simulink model "BMS_Arch_Harness_SIL"  (R2022b)
settings: configuration reference "BMS_Sw_CodeGenConfig" (kept outside this file)
undefined symbols (not defined in the file): BMS_State_Enum
settings Model: DataDictionary=BMS_Arch_DD.sldd  Creator=MAAM  LastModifiedBy=MAAM
settings ConfigSetRef: SourceName=BMS_Sw_CodeGenConfig

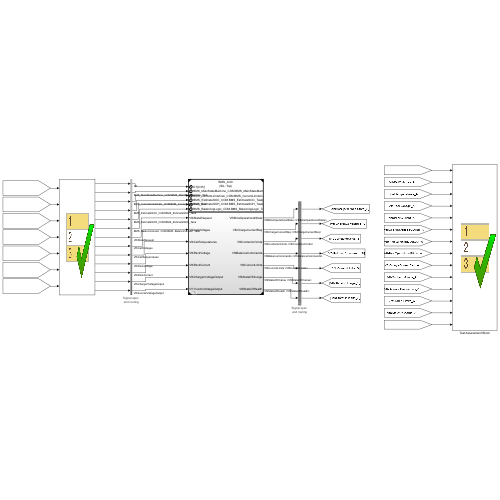
[thumbnail: Simulink's stored preview of the top-level diagram]
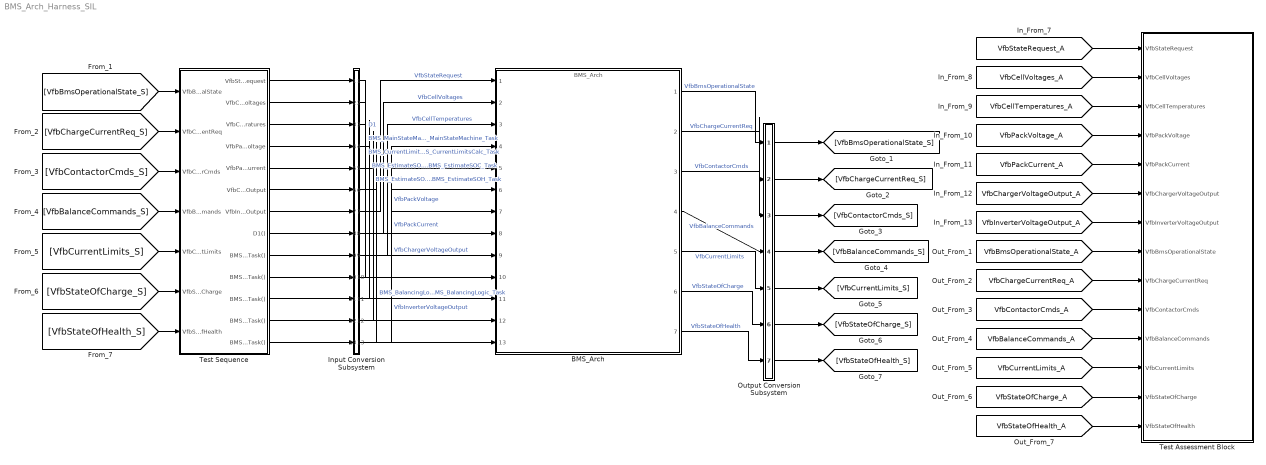
== system BMS_Arch_Harness_SIL ==
  BMS_Arch : ModelReference  ModelNameDialog=BMS_Arch  SimulationMode=Software-in-the-loop (SIL)  ScheduleRates=on  PortDiscreteRates={'',0.05;'BMS_MainStateMachine_COM.BMS_MainStateMachine_Task',0.05;'BMS_CurrentLimitsCalc_COM.BMS_CurrentLimitsCalc_Task',0.1;'BMS_EstimateSOC_COM.BMS_EstimateSOC_Task',0.2;'BMS_EstimateSOH_COM.BMS_EstimateSOH_Task',0.2;'BMS_BalancingLogic_COM.BMS_BalancingLogic_Task',0.25}  CachedPortDiscreteRates={'',0.05;'BMS_MainStateMachine_COM.BMS_MainStateMachine_Task',0.05;'BMS_CurrentLimitsCalc_COM.BMS_CurrentLimitsCalc_Task',0.1;'BMS_EstimateSOC_COM.BMS_EstimateSOC_Task',0.2;'BMS_EstimateSOH_COM.BMS_EstimateSOH_Task',0.2;'BMS_BalancingLogic_COM.BMS_BalancingLogic_Task',0.25}  AutoFillPortDiscreteRates=off  ModelEventPortInfo=P:D1[0.05][0][0],P:BMS_MainStateMachine_COM.BMS_MainStateMachine_Task[0.05][1][0],P:BMS_CurrentLimitsCalc_COM.BMS_CurrentLimitsCalc_Task[0.1][1][0],P:BMS_EstimateSOC_COM.BMS_EstimateSOC_Task[0.2][1][0],P:BMS_EstimateSOH_COM.BMS_EstimateSOH_Task[0.2][1][0],P:BMS_BalancingLogic_COM.BMS_BalancingLogic_Task[0.25][1][0]  CodeInterface=Top model  ModelReferenceVersion=1.62
  Input Conversion Subsystem : Subsystem  Tag=__SLT_ICS__  Description=|
      | Signal spec.
      | and routing
      settings: AttributesFormatString=%<Description>
  Output Conversion Subsystem : Subsystem  Tag=__SLT_OCS__  Description=|
      | Signal spec.
      | and routing
      mask init:
      | ICDictionary = get_param(bdroot, 'DataDictionary');
      | if isempty(ICDictionary)
      |    ICScope = Simulink.data.BaseWorkspace;
      | else
      |    ICScope = Simulink.data.DataDictionary(ICDictionary);
      | end
      | 
      | IC3 = Simulink.Bus.createMATLABStruct('BMS_strContactorCmds', [], [1 1], ICScope);
      settings: AttributesFormatString=%<Description>
  Test Assessment Block : Test Sequence  Tag=__SLT_ASMT__  TreatAsAtomicUnit=on
  Test Sequence : Test Sequence  TreatAsAtomicUnit=on
  wires:
  [VfbStateRequest_A] -> Test Assessment Block/1(VfbStateRequest)
  [VfbCellVoltages_A] -> Test Assessment Block/2(VfbCellVoltages)
  [VfbCellTemperatures_A] -> Test Assessment Block/3(VfbCellTemperatures)
  [VfbPackVoltage_A] -> Test Assessment Block/4(VfbPackVoltage)
  [VfbPackCurrent_A] -> Test Assessment Block/5(VfbPackCurrent)
  [VfbChargerVoltageOutput_A] -> Test Assessment Block/6(VfbChargerVoltageOutput)
  [VfbInverterVoltageOutput_A] -> Test Assessment Block/7(VfbInverterVoltageOutput)
  [VfbBmsOperationalState_A] -> Test Assessment Block/8(VfbBmsOperationalState)
  [VfbChargeCurrentReq_A] -> Test Assessment Block/9(VfbChargeCurrentReq)
  [VfbContactorCmds_A] -> Test Assessment Block/10(VfbContactorCmds)
  [VfbBalanceCommands_A] -> Test Assessment Block/11(VfbBalanceCommands)
  [VfbCurrentLimits_A] -> Test Assessment Block/12(VfbCurrentLimits)
  [VfbStateOfCharge_A] -> Test Assessment Block/13(VfbStateOfCharge)
  [VfbStateOfHealth_A] -> Test Assessment Block/14(VfbStateOfHealth)
  Test Sequence/1(VfbStateRequest) -> Input Conversion Subsystem/1(Inport_1)
  Test Sequence/2(VfbCellVoltages) -> Input Conversion Subsystem/2(Inport_2)
  Test Sequence/3(VfbCellTemperatures) -> Input Conversion Subsystem/3(Inport_3)
  Test Sequence/4(VfbPackVoltage) -> Input Conversion Subsystem/4(Inport_4)
  Test Sequence/5(VfbPackCurrent) -> Input Conversion Subsystem/5(Inport_5)
  Test Sequence/6(VfbChargerVoltageOutput) -> Input Conversion Subsystem/6(Inport_6)
  Test Sequence/7(VfbInverterVoltageOutput) -> Input Conversion Subsystem/7(Inport_7)
  Test Sequence/8(D1()) -> Input Conversion Subsystem/8(Inport_8)
  Test Sequence/9(BMS_MainStateMachine_COMBMS_MainStateMachine_Task()) -> Input Conversion Subsystem/9(Inport_9)
  Test Sequence/10(BMS_CurrentLimitsCalc_COMBMS_CurrentLimitsCalc_Task()) -> Input Conversion Subsystem/10(Inport_10)
  Test Sequence/11(BMS_EstimateSOC_COMBMS_EstimateSOC_Task()) -> Input Conversion Subsystem/11(Inport_11)
  Test Sequence/12(BMS_EstimateSOH_COMBMS_EstimateSOH_Task()) -> Input Conversion Subsystem/12(Inport_12)
  Test Sequence/13(BMS_BalancingLogic_COMBMS_BalancingLogic_Task()) -> Input Conversion Subsystem/13(Inport_13)
  [VfbBmsOperationalState_S] -> Test Sequence/1(VfbBmsOperationalState)
  [VfbChargeCurrentReq_S] -> Test Sequence/2(VfbChargeCurrentReq)
  [VfbContactorCmds_S] -> Test Sequence/3(VfbContactorCmds)
  [VfbBalanceCommands_S] -> Test Sequence/4(VfbBalanceCommands)
  [VfbCurrentLimits_S] -> Test Sequence/5(VfbCurrentLimits)
  [VfbStateOfCharge_S] -> Test Sequence/6(VfbStateOfCharge)
  [VfbStateOfHealth_S] -> Test Sequence/7(VfbStateOfHealth)
  Output Conversion Subsystem/1(Outport_1) -> [VfbBmsOperationalState_S]
  Output Conversion Subsystem/2(Outport_2) -> [VfbChargeCurrentReq_S]
  Output Conversion Subsystem/3(Outport_3) -> [VfbContactorCmds_S]
  Output Conversion Subsystem/4(Outport_4) -> [VfbBalanceCommands_S]
  Output Conversion Subsystem/5(Outport_5) -> [VfbCurrentLimits_S]
  Output Conversion Subsystem/6(Outport_6) -> [VfbStateOfCharge_S]
  Output Conversion Subsystem/7(Outport_7) -> [VfbStateOfHealth_S]
  BMS_Arch/1 -> Output Conversion Subsystem/1(Inport_1)  "VfbBmsOperationalState"
  BMS_Arch/2 -> Output Conversion Subsystem/2(Inport_2)  "VfbChargeCurrentReq"
  BMS_Arch/3 -> Output Conversion Subsystem/3(Inport_3)  "VfbContactorCmds"
  BMS_Arch/4 -> Output Conversion Subsystem/4(Inport_4)  "VfbBalanceCommands"
  BMS_Arch/5 -> Output Conversion Subsystem/5(Inport_5)  "VfbCurrentLimits"
  BMS_Arch/6 -> Output Conversion Subsystem/6(Inport_6)  "VfbStateOfCharge"
  BMS_Arch/7 -> Output Conversion Subsystem/7(Inport_7)  "VfbStateOfHealth"
  Input Conversion Subsystem/1(Outport_1) -> BMS_Arch/8  "D1"
  Input Conversion Subsystem/2(Outport_2) -> BMS_Arch/9  "BMS_MainStateMachine_COM.BMS_MainStateMachine_Task"
  Input Conversion Subsystem/3(Outport_3) -> BMS_Arch/10  "BMS_CurrentLimitsCalc_COM.BMS_CurrentLimitsCalc_Task"
  Input Conversion Subsystem/4(Outport_4) -> BMS_Arch/11  "BMS_EstimateSOC_COM.BMS_EstimateSOC_Task"
  Input Conversion Subsystem/5(Outport_5) -> BMS_Arch/12  "BMS_EstimateSOH_COM.BMS_EstimateSOH_Task"
  Input Conversion Subsystem/6(Outport_6) -> BMS_Arch/13  "BMS_BalancingLogic_COM.BMS_BalancingLogic_Task"
  Input Conversion Subsystem/7(Outport_7) -> BMS_Arch/1  "VfbStateRequest"
  Input Conversion Subsystem/8(Outport_8) -> BMS_Arch/2  "VfbCellVoltages"
  Input Conversion Subsystem/9(Outport_9) -> BMS_Arch/3  "VfbCellTemperatures"
  Input Conversion Subsystem/10(Outport_10) -> BMS_Arch/4  "VfbPackVoltage"
  Input Conversion Subsystem/11(Outport_11) -> BMS_Arch/5  "VfbPackCurrent"
  Input Conversion Subsystem/12(Outport_12) -> BMS_Arch/6  "VfbChargerVoltageOutput"
  Input Conversion Subsystem/13(Outport_13) -> BMS_Arch/7  "VfbInverterVoltageOutput"

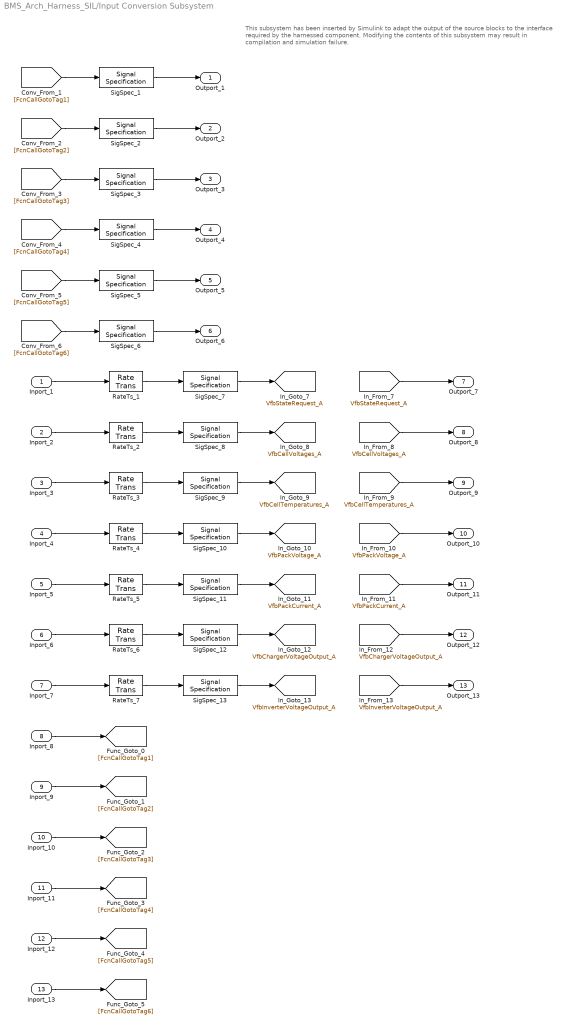
== system BMS_Arch_Harness_SIL/Input Conversion Subsystem ==
  note: This subsystem has been inserted by Simulink to adapt the output of the source blocks to the interface required by the harnessed component.
      |  Modifying the contents of this subsystem may result in compilation and simulation failure.
  Inport_1 : Inport
  Inport_2 : Inport  Port=2
  Inport_3 : Inport  Port=3
  Inport_4 : Inport  Port=4
  Inport_5 : Inport  Port=5
  Inport_6 : Inport  Port=6
  Inport_7 : Inport  Port=7
  Inport_8 : Inport  Port=8
  Inport_9 : Inport  Port=9
  Inport_10 : Inport  Port=10
  Inport_11 : Inport  Port=11
  Inport_12 : Inport  Port=12
  Inport_13 : Inport  Port=13
  RateTs_1 : RateTransition  InitialCondition=BMS_State_Enum.BMS_Standby
  RateTs_{2..7} (6 alike) : RateTransition
  SigSpec_{1..6} (6 alike) : SignalSpecification
  SigSpec_{8,10,12..13} (4 alike) : SignalSpecification  OutDataTypeStr=single  Unit=V  Dimensions=[1]
  SigSpec_11 : SignalSpecification  OutDataTypeStr=single  Unit=A  Dimensions=[1]
  SigSpec_7 : SignalSpecification  OutDataTypeStr=Enum: BMS_State_Enum  Dimensions=[1]
  SigSpec_9 : SignalSpecification  OutDataTypeStr=single  Unit=°C  Dimensions=[1]
  Outport_1 : Outport
  Outport_2 : Outport  Port=2
  Outport_3 : Outport  Port=3
  Outport_4 : Outport  Port=4
  Outport_5 : Outport  Port=5
  Outport_6 : Outport  Port=6
  Outport_7 : Outport  Port=7
  Outport_8 : Outport  Port=8
  Outport_9 : Outport  Port=9
  Outport_10 : Outport  Port=10
  Outport_11 : Outport  Port=11
  Outport_12 : Outport  Port=12
  Outport_13 : Outport  Port=13
  tag scope: VfbCellTemperatures_A=global, VfbCellVoltages_A=global, VfbChargerVoltageOutput_A=global, VfbInverterVoltageOutput_A=global, VfbPackCurrent_A=global, VfbPackVoltage_A=global, VfbStateRequest_A=global
  wires:
  SigSpec_1/1 -> Outport_1/1
  [FcnCallGotoTag1] -> SigSpec_1/1
  SigSpec_2/1 -> Outport_2/1
  [FcnCallGotoTag2] -> SigSpec_2/1
  SigSpec_3/1 -> Outport_3/1
  [FcnCallGotoTag3] -> SigSpec_3/1
  SigSpec_4/1 -> Outport_4/1
  [FcnCallGotoTag4] -> SigSpec_4/1
  SigSpec_5/1 -> Outport_5/1
  [FcnCallGotoTag5] -> SigSpec_5/1
  SigSpec_6/1 -> Outport_6/1
  [FcnCallGotoTag6] -> SigSpec_6/1
  [VfbStateRequest_A] -> Outport_7/1
  SigSpec_7/1 -> [VfbStateRequest_A]
  RateTs_1/1 -> SigSpec_7/1
  Inport_1/1 -> RateTs_1/1
  [VfbCellVoltages_A] -> Outport_8/1
  SigSpec_8/1 -> [VfbCellVoltages_A]
  RateTs_2/1 -> SigSpec_8/1
  Inport_2/1 -> RateTs_2/1
  [VfbCellTemperatures_A] -> Outport_9/1
  SigSpec_9/1 -> [VfbCellTemperatures_A]
  RateTs_3/1 -> SigSpec_9/1
  Inport_3/1 -> RateTs_3/1
  [VfbPackVoltage_A] -> Outport_10/1
  SigSpec_10/1 -> [VfbPackVoltage_A]
  RateTs_4/1 -> SigSpec_10/1
  Inport_4/1 -> RateTs_4/1
  [VfbPackCurrent_A] -> Outport_11/1
  SigSpec_11/1 -> [VfbPackCurrent_A]
  RateTs_5/1 -> SigSpec_11/1
  Inport_5/1 -> RateTs_5/1
  [VfbChargerVoltageOutput_A] -> Outport_12/1
  SigSpec_12/1 -> [VfbChargerVoltageOutput_A]
  RateTs_6/1 -> SigSpec_12/1
  Inport_6/1 -> RateTs_6/1
  [VfbInverterVoltageOutput_A] -> Outport_13/1
  SigSpec_13/1 -> [VfbInverterVoltageOutput_A]
  RateTs_7/1 -> SigSpec_13/1
  Inport_7/1 -> RateTs_7/1
  Inport_8/1 -> [FcnCallGotoTag1]
  Inport_9/1 -> [FcnCallGotoTag2]
  Inport_10/1 -> [FcnCallGotoTag3]
  Inport_11/1 -> [FcnCallGotoTag4]
  Inport_12/1 -> [FcnCallGotoTag5]
  Inport_13/1 -> [FcnCallGotoTag6]

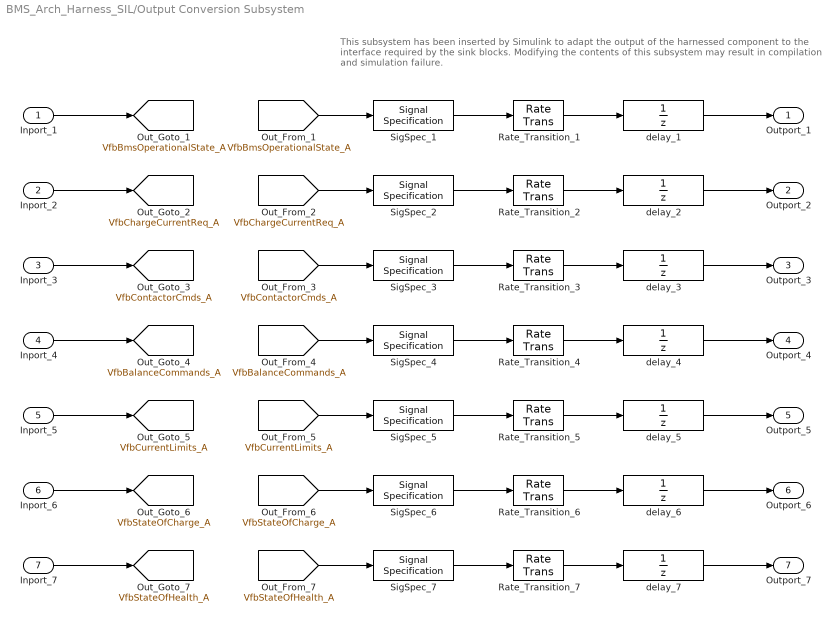
== system BMS_Arch_Harness_SIL/Output Conversion Subsystem ==
  note: This subsystem has been inserted by Simulink to adapt the output of the harnessed component to the interface required by the sink blocks.
      |  Modifying the contents of this subsystem may result in compilation and simulation failure.
  Inport_1 : Inport
  Inport_2 : Inport  Port=2
  Inport_3 : Inport  Port=3
  Inport_4 : Inport  Port=4
  Inport_5 : Inport  Port=5
  Inport_6 : Inport  Port=6
  Inport_7 : Inport  Port=7
  Rate_Transition_1 : RateTransition  InitialCondition=BMS_State_Enum.BMS_Standby  OutPortSampleTimeOpt=Inherit
  Rate_Transition_{2..7} (6 alike) : RateTransition  OutPortSampleTimeOpt=Inherit
  SigSpec_1 : SignalSpecification  OutDataTypeStr=Enum: BMS_State_Enum  Dimensions=[1]
  SigSpec_2 : SignalSpecification  OutDataTypeStr=single  Unit=A  Dimensions=[1]
  SigSpec_3 : SignalSpecification  OutDataTypeStr=Bus: BMS_strContactorCmds  Dimensions=[1]  BusOutputAsStruct=on
  SigSpec_4 : SignalSpecification  OutDataTypeStr=boolean  Dimensions=[1]
  SigSpec_5 : SignalSpecification  OutDataTypeStr=single  Unit=A  Dimensions=[2]
  SigSpec_6 : SignalSpecification  OutDataTypeStr=single  Unit=%  Dimensions=[3]
  SigSpec_7 : SignalSpecification  OutDataTypeStr=single  Unit=%  Dimensions=[3]
  delay_1 : UnitDelay  InitialCondition=BMS_State_Enum.BMS_Standby  SampleTime=-1
  delay_{2,4..7} (5 alike) : UnitDelay  SampleTime=-1
  delay_3 : UnitDelay  InitialCondition=IC3  SampleTime=-1
  Outport_1 : Outport
  Outport_2 : Outport  Port=2
  Outport_3 : Outport  Port=3
  Outport_4 : Outport  Port=4
  Outport_5 : Outport  Port=5
  Outport_6 : Outport  Port=6
  Outport_7 : Outport  Port=7
  tag scope: VfbBalanceCommands_A=global, VfbBmsOperationalState_A=global, VfbChargeCurrentReq_A=global, VfbContactorCmds_A=global, VfbCurrentLimits_A=global, VfbStateOfCharge_A=global, VfbStateOfHealth_A=global
  wires:
  Inport_1/1 -> [VfbBmsOperationalState_A]
  [VfbBmsOperationalState_A] -> SigSpec_1/1
  SigSpec_1/1 -> Rate_Transition_1/1
  Rate_Transition_1/1 -> delay_1/1
  delay_1/1 -> Outport_1/1
  Inport_2/1 -> [VfbChargeCurrentReq_A]
  [VfbChargeCurrentReq_A] -> SigSpec_2/1
  SigSpec_2/1 -> Rate_Transition_2/1
  Rate_Transition_2/1 -> delay_2/1
  delay_2/1 -> Outport_2/1
  Inport_3/1 -> [VfbContactorCmds_A]
  [VfbContactorCmds_A] -> SigSpec_3/1
  SigSpec_3/1 -> Rate_Transition_3/1
  Rate_Transition_3/1 -> delay_3/1
  delay_3/1 -> Outport_3/1
  Inport_4/1 -> [VfbBalanceCommands_A]
  [VfbBalanceCommands_A] -> SigSpec_4/1
  SigSpec_4/1 -> Rate_Transition_4/1
  Rate_Transition_4/1 -> delay_4/1
  delay_4/1 -> Outport_4/1
  Inport_5/1 -> [VfbCurrentLimits_A]
  [VfbCurrentLimits_A] -> SigSpec_5/1
  SigSpec_5/1 -> Rate_Transition_5/1
  Rate_Transition_5/1 -> delay_5/1
  delay_5/1 -> Outport_5/1
  Inport_6/1 -> [VfbStateOfCharge_A]
  [VfbStateOfCharge_A] -> SigSpec_6/1
  SigSpec_6/1 -> Rate_Transition_6/1
  Rate_Transition_6/1 -> delay_6/1
  delay_6/1 -> Outport_6/1
  Inport_7/1 -> [VfbStateOfHealth_A]
  [VfbStateOfHealth_A] -> SigSpec_7/1
  SigSpec_7/1 -> Rate_Transition_7/1
  Rate_Transition_7/1 -> delay_7/1
  delay_7/1 -> Outport_7/1

== stateflow chart BMS_Arch_Harness_SIL/Test Assessment Block ==
  state Run
    state step_1_1
    state step_1_2
    (default) -> (junction 22)
    Run -> (junction 22)
    (junction 22) -> (junction 23) [order 1] : [t < 5
        | ]
    (junction 23) -> step_1_1 [order 1] : [~in(Run.step_1_1)]
    (junction 23) -> (junction 26) [order 2]
    (junction 31) -> (junction 32)
    (junction 32) -> step_1_2 [order 1] : [~in(Run.step_1_2)]
    (junction 32) -> (junction 35) [order 2]
    (junction 22) -> (junction 31) [order 2]
  (default) -> Run
  data: VfbStateRequest input Enum: BMS_State_Enum size=[1]; VfbCellVoltages input single size=[1]; VfbCellTemperatures input single size=[1]; VfbPackVoltage input single size=[1]; VfbPackCurrent input single size=[1]; VfbChargerVoltageOutput input single size=[1]; VfbInverterVoltageOutput input single size=[1]; VfbBmsOperationalState input Enum: BMS_State_Enum size=[1]; VfbChargeCurrentReq input single size=[1]; VfbContactorCmds input Bus: BMS_strContactorCmds size=[1]; VfbBalanceCommands input boolean size=[1]; VfbCurrentLimits input single size=[2]; VfbStateOfCharge input single size=[3]; VfbStateOfHealth input single size=[3]

== stateflow chart BMS_Arch_Harness_SIL/Test Sequence ==
  settings: updateMethod=DISCRETE  sampleTime=0.05
  state Run
    %% Initialize data outputs.
    VfbStateRequest = BMS_State_Enum.BMS_Standby;
    VfbCellVoltages = single(0);
    VfbCellTemperatures = single(0);
    VfbPackVoltage = single(0);
    VfbPackCurrent = single(0);
    VfbChargerVoltageOutput = single(0);
    VfbInverterVoltageOutput = single(0);
    send(D1);
    send(BMS_MainStateMachine_COMBMS_MainStateMachine_Task);
    if t == 0 || every(2, tick)
    send(BMS_CurrentLimitsCalc_COMBMS_CurrentLimitsCalc_Task);
    end
    if t == 0 || every(4, tick)
    send(BMS_EstimateSOC_COMBMS_EstimateSOC_Task);
    end
    if t == 0 || every(4, tick)
    send(BMS_EstimateSOH_COMBMS_EstimateSOH_Task);
    end
    if t == 0 || every(5, tick)
    send(BMS_BalancingLogic_COMBMS_BalancingLogic_Task);
    end
  (default) -> Run
  data: VfbBmsOperationalState input Enum: BMS_State_Enum size=[1]; VfbChargeCurrentReq input single size=[1]; VfbContactorCmds input Bus: BMS_strContactorCmds size=[1]; VfbBalanceCommands input boolean size=[1]; VfbCurrentLimits input single size=[2]; VfbStateOfCharge input single size=[3]; VfbStateOfHealth input single size=[3]; VfbStateRequest output Enum: BMS_State_Enum size=[1]; VfbCellVoltages output single size=[1]; VfbCellTemperatures output single size=[1]; VfbPackVoltage output single size=[1]; VfbPackCurrent output single size=[1]; VfbChargerVoltageOutput output single size=[1]; VfbInverterVoltageOutput output single size=[1]
  events: D1 output FUNCTION_CALL_EVENT; BMS_MainStateMachine_COMBMS_MainStateMachine_Task output FUNCTION_CALL_EVENT; BMS_CurrentLimitsCalc_COMBMS_CurrentLimitsCalc_Task output FUNCTION_CALL_EVENT; BMS_EstimateSOC_COMBMS_EstimateSOC_Task output FUNCTION_CALL_EVENT; BMS_EstimateSOH_COMBMS_EstimateSOH_Task output FUNCTION_CALL_EVENT; BMS_BalancingLogic_COMBMS_BalancingLogic_Task output FUNCTION_CALL_EVENT
